simulink model "MotorPlant_23_lab2_part_e"  (R2019b)
settings: Solver=FixedStepAuto  StartTime=0.0  StopTime=2  FixedStep=0.001  RelTol=1e-3
settings Model: Creator=cmcaradi  LastModifiedBy=Laura

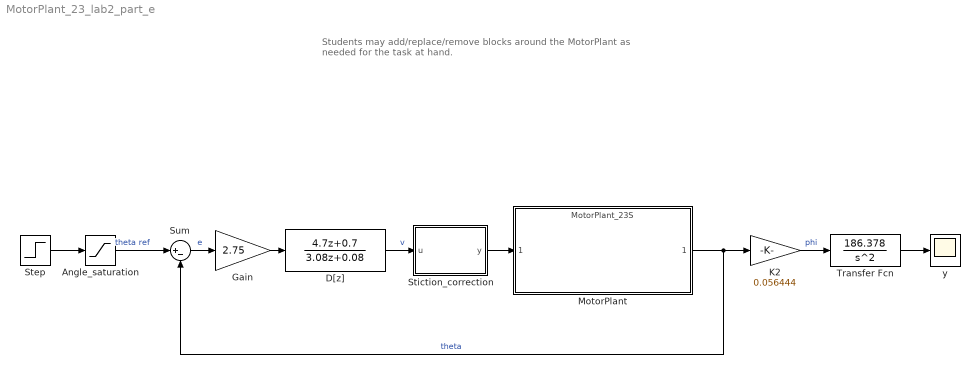
== system MotorPlant_23_lab2_part_e ==
  note: Students may add/replace/remove blocks around the
      | MotorPlant as needed for the task at hand.
  Angle_saturation : Saturate  UpperLimit=0.7  LowerLimit=-0.7
  D[z] : DiscreteTransferFcn  Numerator=[4.7 0.7]  Denominator=[3.08 0.08]  SampleTime=0.03
  Gain : Gain  Gain=2.75
  K2 : Gain  Gain=0.056444
  MotorPlant : ModelReference  ModelNameDialog=MotorPlant_23S  ModelReferenceVersion=1.41  CopyOfModelProtected=on
  Step : Step  Before=-0.7  After=0.7  SampleTime=0
  Stiction_correction : MATLAB Function  TreatAsAtomicUnit=on
  Sum : Sum  Inputs=|+-
  Transfer Fcn : TransferFcn  Numerator=[186.378]  Denominator=[1 0 0]
  y : Scope
  wires:
  MotorPlant/1 -> K2/1, Sum/2  "theta"
  Angle_saturation/1 -> Sum/1  "theta ref"
  Stiction_correction/1(y) -> MotorPlant/1
  Step/1 -> Angle_saturation/1
  Gain/1 -> D[z]/1
  Sum/1 -> Gain/1  "e"
  D[z]/1 -> Stiction_correction/1(u)  "v"
  K2/1 -> Transfer Fcn/1  "phi"
  Transfer Fcn/1 -> y/1

== matlab function MotorPlant_23_lab2_part_e/Stiction_correction ==
  data: u input; y output
function y = fcn(u)

a = -0.48;
b = 0.50;

if u < b && u > 0
    y = u + b;
elseif u > a && u < 0
    y = u + a;
else
    y = u;

end
